simulink model "test"  (R2017a)
settings: Solver=VariableStepAuto  StartTime=0.0  StopTime=10.0  RelTol=1e-3
model workspace: external: MAT-File C:\Users\calvinv\Google Drive\code\Matlab\QuadSim\Simulink\parameters\param.mat (data not in the file)
settings Model: Creator=calvin  LastModifiedBy=calvinv

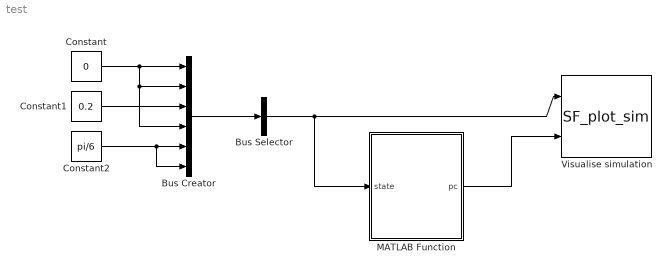
== system test ==
  Bus Creator : BusCreator  Inputs=6
  Bus Selector : BusSelector  OutputSignals=signal1,signal2,signal3,signal4,signal5,signal6  OutputAsBus=on
  Constant : Constant  Value=0
  Constant1 : Constant  Value=0.2
  Constant2 : Constant  Value=pi/6
  MATLAB Function : MATLAB Function  TreatAsAtomicUnit=on
  Visualise simulation : M-S-Function  FunctionName=SF_plot_sim  Parameters=quad
  wires:
  Bus Selector/1 -> Visualise simulation/1, MATLAB Function/1(state)
  Bus Creator/1 -> Bus Selector/1
  Constant/1 -> Bus Creator/2, Bus Creator/4, Bus Creator/1
  MATLAB Function/1(pc) -> Visualise simulation/2
  Constant1/1 -> Bus Creator/3
  Constant2/1 -> Bus Creator/6, Bus Creator/5

== matlab function test/MATLAB Function ==
  data: state input; pc output
%% need another and condition inside wall check


function pc = lidar_scan_gen(state)

%% init
tunnel_r = 1.5;
tunnel_l = 6; % tunnel length;

a = -135:0.25:135; % lidar FOV is 270 deg

a = a .* pi/180;

pc = zeros(length(a)+5, 3);
temp = zeros(length(a), 3);

z_ceiling = 2 * tunnel_r;
z_ground = 0;

wall_left = -tunnel_r;
wall_right = tunnel_r;

pos_x = state(1);
pos_y = state(2);
pos_z = state(3);
phi = state(4);
the = state(5);
psi = state(6);

%% checking intersection 
np = 1;
c = 1;
oline = zeros(5,3);

for m = 1:length(a)
    
    angle = [phi the psi];
    
    % generate line point
    r = 20*tunnel_r;
    p = [0 r*sin(a(m)) r*cos(a(m))]';

    pos = [pos_x pos_y pos_z]; % position of the quad
    
    p = Rzyx(angle) * p + pos';    % apply rotation
    
    % wall planes - top right bot left
    n = [0 0 1;0 1 0;0 0 1;0 -1 0];
    wall0 = [0 0 z_ceiling;0 wall_right 0;0 0 z_ground;0 wall_left 0];
    
    for b = 1:4
        [p_wall,check] = plane_line_intersect(n(b, :), wall0(b, :) ,pos ,p');

        if check == 1
            if round(p_wall(2)*1e10)/1e10 > wall_right || round(p_wall(2)*1e10)/1e10 < wall_left
                continue;
            elseif round(p_wall(3)*1e10)/1e10 > z_ceiling || round(p_wall(3)*1e10)/1e10 < z_ground   
                continue;
            else
                break;
            end
        end
    end
    
    % oline is for plotting the centre lines
    
    if m == 1 || m == 1081 || m == 1080/2 || m == 180 || m == 1081-180
        oline(c,:) = p_wall;
        c = c + 1;
    end
    
    lidar_noise = [0 50 - randi(100,1) 50-randi(100,1)]./1000 ; % +/- 50mm noise
    
    temp(np,:) = p_wall + lidar_noise;
    np = np + 1;
end

pc = [oline;temp];

end
